simulink model "rov_property"  (Simulink 6.0)
settings: Solver=ode45  StartTime=0.0  StopTime=20  RelTol=1e-5
undefined symbols (not defined in the file): B, DQ, DQL, I, m, M, Ma, MaU, rg, T, uc1, uc2, uc3, uc4, W, xb, xg, Xudot, yb, yg, Yvdot, zb, zg, Zwdot
libraries: simulink x18, rov_design_analysis x5
(part 1 of 2)
settings Model: LastModifiedBy=c chin

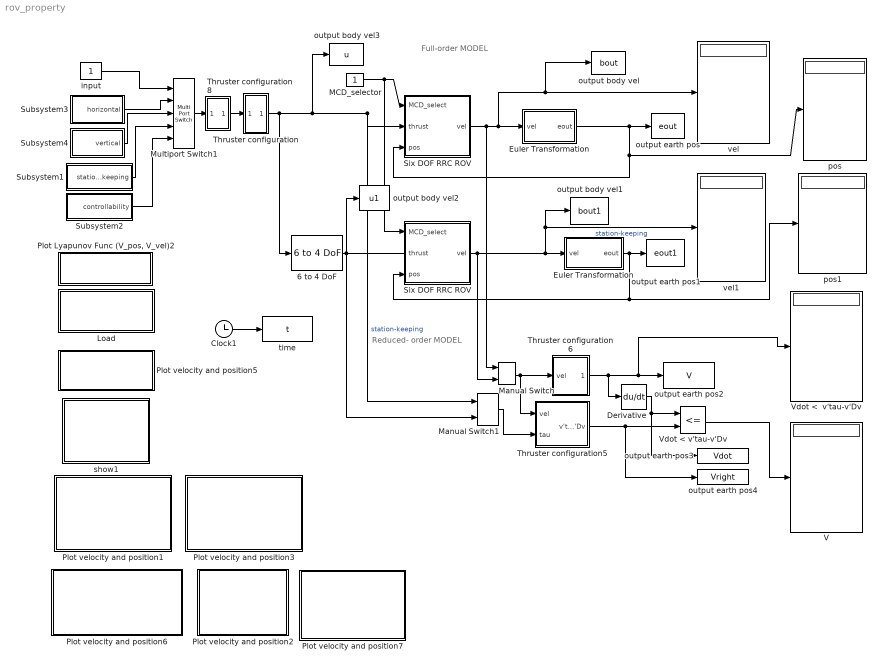
== system rov_property ==
  note: Full-order MODEL
  note: Reduced- order
      | MODEL
  " Load  " : Subsystem  AncestorBlock=|
      | rov_design_analysis/ROV Controller
      | Design
      | Applications/ Load RRCROV2 parameters
      settings: OpenFcn=|
      | clear
      | clc
      | cd c:\Matlab7\toolbox\rov_design_analysis\\mat_file ;
      | load rrcrovf;
      | cd c:\Matlab7\toolbox\rov_design_analysis\hybrid ;
      | uc1=70;uc2=70;uc3=70;uc4=70;
      mask Display: disp('Load the\n RRCROV2\n parameters')
  " Six DOF RRC ROV  " : Subsystem
      mask Display:
      | disp('ROV')
      | image(imread('/rov_design_analysis/fig/ROVRRC2.jpg'));
      | color('white');port_label('input',2,'thrust')
      | color('white');port_label('input',1,'MCD_select')
      | color('white');port_label('input',3,'pos')
      | color('white');port_label('output',1,'vel')
      | color('white');port_label('output',2,'Inv_MC')
  " Six DOF RRC ROV   " : Subsystem
      mask Display:
      | disp('ROV')
      | image(imread('/rov_design_analysis/fig/ROVRRC2.jpg'));
      | color('white');port_label('input',2,'thrust')
      | color('white');port_label('input',1,'MCD_select')
      | color('white');port_label('input',3,'pos')
      | color('white');port_label('output',1,'vel')
      | color('white');port_label('output',2,'Inv_MC')
  6 to 4 DoF : rov_design_analysis/Utilities/6 to 4 DoF
  Clock1 : Clock
      settings: Decimation=10
  Derivative : Derivative
  Euler Transformation : Subsystem  AncestorBlock=rov_design_analysis/Scope Utilities/Euler Transformation
  "Euler Transformation  " : Subsystem  AncestorBlock=rov_design_analysis/Scope Utilities/Euler Transformation
  MCD_selector : Constant
  Manual Switch : simulink/Signal Routing/Manual Switch  sw=0  action=0
  Manual Switch1 : simulink/Signal Routing/Manual Switch  sw=0  action=0
  Multiport Switch1 : MultiPortSwitch
  "Plot Lyapunov Func (V_pos, V_vel)2" : Subsystem  AncestorBlock=|
      | rov_design_analysis/ROV Controller
      | Design
      | Applications/Plot velocity and position
      settings: OpenFcn=|
      | clc
      | close all
      mask Display: disp('Close All Figure')
  Plot velocity and position1 : Subsystem  AncestorBlock=|
      | rov_design_analysis/ROV Controller
      | Design
      | Applications/Plot velocity and position
      settings: OpenFcn=|
      | clc
      | cd c:\Matlab7\toolbox\rov_design_analysis\hybrid
      | run nonlin_unique
      mask Display: disp('2a) Double-click \n to \n check \n Uniqueness/Existence \n & Continuous \n (Station)')
  Plot velocity and position2 : Subsystem  AncestorBlock=|
      | rov_design_analysis/ROV Controller
      | Design
      | Applications/Plot velocity and position
      settings: OpenFcn=|
      | clc
      | cd C:\Matlab7\toolbox\rov_design_analysis\nonlin_analysis
      | run control_analy
      mask Display: disp('3b) Double-click \n to \n check \n controllability ')
  Plot velocity and position3 : Subsystem  AncestorBlock=|
      | rov_design_analysis/ROV Controller
      | Design
      | Applications/Plot velocity and position
      settings: OpenFcn=|
      | clc
      | cd c:\Matlab7\toolbox\rov_design_analysis\hybrid
      | run nonlin_unique_plane
      mask Display: disp('2b) Double-click \n to \n check \n Uniqueness/Existence \n & Continuous \n (Vert/Hort)')
  Plot velocity and position5 : Subsystem  AncestorBlock=|
      | rov_design_analysis/ROV Controller
      | Design
      | Applications/Plot velocity and position
      settings: OpenFcn=|
      | clc
      | cd c:\Matlab7\toolbox\rov_design_analysis\hybrid
      | sim('rov_property')
      mask Display: disp('Run  SIMULINK')
  Plot velocity and position6 : Subsystem  AncestorBlock=|
      | rov_design_analysis/ROV Controller
      | Design
      | Applications/Plot velocity and position
      settings: OpenFcn=|
      | clc
      | cd C:\Matlab7\toolbox\rov_design_analysis\hybrid
      | run controllable_property
      mask Display: disp('3a) Double-click \n to \n check \n unactuated/actuated mode')
  Plot velocity and position7 : Subsystem  AncestorBlock=|
      | rov_design_analysis/ROV Controller
      | Design
      | Applications/Plot velocity and position
      settings: OpenFcn=|
      | clc
      | cd C:\Matlab7\toolbox\rov_design_analysis\hybrid
      | open controllable_property
      mask Display: disp('3c) Open \n controllability mdl')
  Subsystem1 : Subsystem
  Subsystem2 : Subsystem
  Subsystem3 : Subsystem
  Subsystem4 : Subsystem
  Thruster configuration : Subsystem
      mask Display: disp('T')
  Thruster configuration5 : Subsystem
  Thruster configuration6 : Subsystem
      mask Display:
      | disp('')
      | color('black');port_label('input',1,'vel')
      | color('black');port_label('output',1,'V')
  Thruster configuration8 : Subsystem  AncestorBlock=|
      | rov_design_analysis/ROV Controller
      | Design
      | Applications/1. Heading autopilot/Thruster
      | configuration
      mask Display: disp('F_T')
  "V " : Display
  "Vdot <  v'tau-v'Dv " : Display
  Vdot < v'tau-v'Dv : RelationalOperator  Operator=<=  LogicOutDataTypeMode=Boolean
  "input " : Constant
  output body vel : ToWorkspace  VariableName=bout  SampleTime=1  SaveFormat=Array
  output body vel1 : ToWorkspace  VariableName=bout1  SampleTime=1  SaveFormat=Array
  output body vel2 : ToWorkspace  VariableName=u1  SampleTime=1  SaveFormat=Array
  output body vel3 : ToWorkspace  VariableName=u  SampleTime=1  SaveFormat=Array
  output earth pos : ToWorkspace  VariableName=eout  SampleTime=1  SaveFormat=Array
  output earth pos1 : ToWorkspace  VariableName=eout1  SampleTime=1  SaveFormat=Array
  output earth pos2 : ToWorkspace  VariableName=V  SampleTime=1  SaveFormat=Array
  output earth pos3 : ToWorkspace  VariableName=Vdot  SampleTime=1  SaveFormat=Array
  output earth pos4 : ToWorkspace  VariableName=Vright  SampleTime=1  SaveFormat=Array
  pos : Display
  pos1 : Display
  show1 : Subsystem  AncestorBlock=|
      | rov_design_analysis/ROV Controller
      | Design
      | Applications/ Load RRCROV2 parameters
      settings: OpenFcn=|
      | clc
      | cd  c:\Matlab7\toolbox\rov_design_analysis\m_file
      | run state_coupling
      mask Display: disp('1) Open \n state-coupling \n analysis')
  time : ToWorkspace  VariableName=t  SampleTime=1  SaveFormat=Array
  vel : Display
  vel1 : Display
  wires:
  Thruster configuration/1(output force) -> output body vel3/1, Manual Switch1/1, " Six DOF RRC ROV   "/2("thrust "), 6 to 4 DoF/1  "station-keeping"
  Clock1/1 -> time/1
  Subsystem4/1(vertical) -> Multiport Switch1/3
  Subsystem3/1(horizontal) -> Multiport Switch1/2
  "input "/1 -> Multiport Switch1/1
  Subsystem1/1(station-keeping) -> Multiport Switch1/4
  Multiport Switch1/1 -> Thruster configuration8/1(input velocity)
  Thruster configuration8/1(output force) -> Thruster configuration/1(input velocity)
  Euler Transformation/1(eout) -> output earth pos/1, pos/1, " Six DOF RRC ROV   "/3("pos ")
  " Six DOF RRC ROV   "/1(vel) -> Euler Transformation/1(vel), output body vel/1, vel/1, Manual Switch/1
  Thruster configuration6/1(energy) -> Derivative/1, output earth pos2/1, "Vdot <  v'tau-v'Dv "/1
  Derivative/1 -> Vdot < v'tau-v'Dv/1, output earth pos3/1
  Thruster configuration5/1(v'tau-v'Dv) -> Vdot < v'tau-v'Dv/2, output earth pos4/1
  Manual Switch/1 -> Thruster configuration6/1(vel), Thruster configuration5/1(vel)
  Manual Switch1/1 -> Thruster configuration5/2(tau)
  Vdot < v'tau-v'Dv/1 -> "V "/1
  " Six DOF RRC ROV  "/1(vel) -> Manual Switch/2, "Euler Transformation  "/1(vel), output body vel1/1, vel1/1  "station-keeping"
  "Euler Transformation  "/1(eout) -> output earth pos1/1, pos1/1, " Six DOF RRC ROV  "/3("pos ")
  6 to 4 DoF/1 -> Manual Switch1/2, " Six DOF RRC ROV  "/2("thrust "), output body vel2/1
  MCD_selector/1 -> " Six DOF RRC ROV   "/1(MCD_select), " Six DOF RRC ROV  "/1(MCD_select)
  Subsystem2/1(controllability) -> Multiport Switch1/5

== system rov_property/ Load   ==

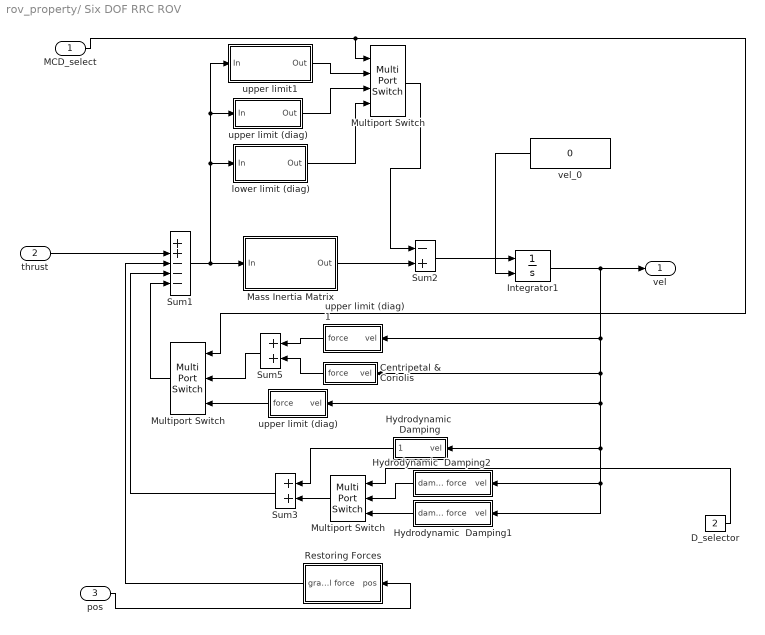
== system rov_property/ Six DOF RRC ROV   ==
  MCD_select : Inport  Port=1  LatchInput=off
  "thrust " : Inport  Port=2  LatchInput=off
  "pos " : Inport  Port=3  LatchInput=off
  Centripetal & Coriolis : Subsystem  Orientation=left  AncestorBlock=rov_design_analysis/ROV Models/1. Six DOF RRC ROV II/Centripetal & Coriolis
      mask Display: disp('C')
  D_selector : Constant  Value=2
  Hydrodynamic  Damping : Subsystem  Orientation=left
      mask Display: disp('D')
  Hydrodynamic  Damping1 : Subsystem  Orientation=left
      mask Display: disp('perturb \nDamping')
  Hydrodynamic  Damping2 : Subsystem  Orientation=left
      mask Display: disp('Zero Perturb')
  Integrator1 : Integrator  InitialConditionSource=external
  Mass Inertia Matrix : Subsystem
      mask Display: disp('inv(MRB+MA)')
  Multiport Switch : MultiPortSwitch  Inputs=3
  "Multiport Switch  " : MultiPortSwitch  Orientation=left  Inputs=2
  "Multiport Switch    " : MultiPortSwitch  Orientation=left  Inputs=2
  Restoring Forces : Subsystem  Orientation=left
      mask Display: disp('Restoring\nForce')
  Sum1 : Sum  Inputs=++---  SaturateOnIntegerOverflow=on  InputSameDT=on
  Sum2 : Sum  Inputs=-+  SaturateOnIntegerOverflow=on  InputSameDT=on
  Sum3 : Sum  Orientation=left  SaturateOnIntegerOverflow=on  InputSameDT=on
  Sum5 : Sum  Orientation=left  SaturateOnIntegerOverflow=on  InputSameDT=on
  lower limit (diag) : Subsystem
      mask Display: disp('Perturb MA')
  upper limit (diag) : Subsystem
      mask Display: disp('Perturb MA')
  "upper limit (diag)   " : Subsystem  Orientation=left
      mask Display: disp('Perturb CA')
  upper limit (diag)   1 : Subsystem  Orientation=left
      mask Display: disp('CA')
  upper limit1 : Subsystem
      mask Display: disp('Zero Perturb')
  vel_0 : Constant  Orientation=left  Value=0  OutDataTypeMode=double
  vel : Outport
  wires:
  Restoring Forces/1(gravitational force) -> Sum1/3
  "thrust "/1 -> Sum1/2
  Sum1/1 -> Mass Inertia Matrix/1(In), upper limit1/1(In), upper limit (diag)/1(In), lower limit (diag)/1(In)
  "Multiport Switch  "/1 -> Sum1/5
  "pos "/1 -> Restoring Forces/1(pos)
  Mass Inertia Matrix/1(Out) -> Sum2/2
  upper limit1/1(Out) -> Multiport Switch/2
  upper limit (diag)/1(Out) -> Multiport Switch/3
  lower limit (diag)/1(Out) -> Multiport Switch/4
  Multiport Switch/1 -> Sum2/1
  "upper limit (diag)   "/1(force) -> "Multiport Switch  "/3
  Sum5/1 -> "Multiport Switch  "/2
  Hydrodynamic  Damping1/1(damping force) -> "Multiport Switch    "/3
  Hydrodynamic  Damping2/1(damping force) -> "Multiport Switch    "/2
  Sum3/1 -> Sum1/4
  "Multiport Switch    "/1 -> Sum3/2
  Hydrodynamic  Damping/1(damping force) -> Sum3/1
  MCD_select/1 -> Multiport Switch/1, "Multiport Switch  "/1
  upper limit (diag)   1/1(force) -> Sum5/1
  Centripetal & Coriolis/1(force) -> Sum5/2
  Sum2/1 -> Integrator1/1
  Integrator1/1 -> vel/1, upper limit (diag)   1/1(vel), Centripetal & Coriolis/1(vel), Hydrodynamic  Damping/1(vel), Hydrodynamic  Damping1/1(vel), Hydrodynamic  Damping2/1(vel), "upper limit (diag)   "/1(vel)
  vel_0/1 -> Integrator1/2
  D_selector/1 -> "Multiport Switch    "/1

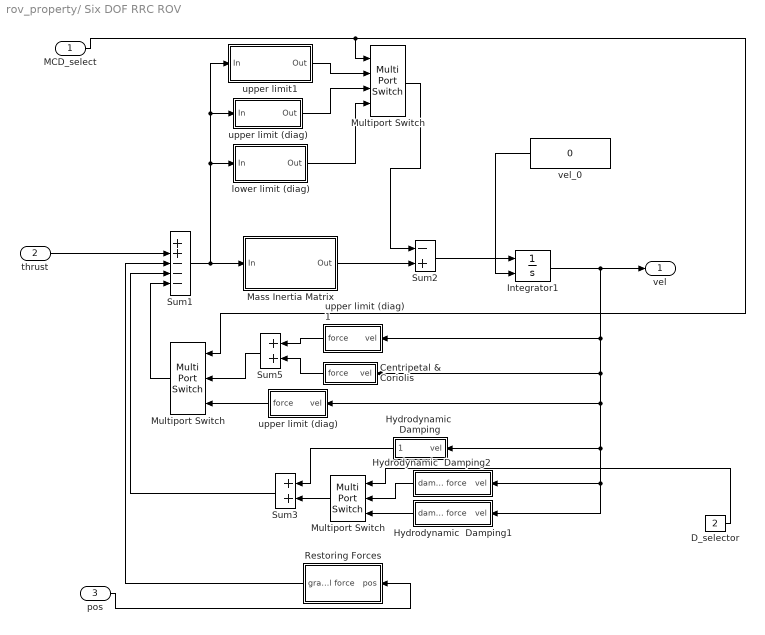
== system rov_property/ Six DOF RRC ROV    ==
  MCD_select : Inport  Port=1  LatchInput=off
  "thrust " : Inport  Port=2  LatchInput=off
  "pos " : Inport  Port=3  LatchInput=off
  Centripetal & Coriolis : Subsystem  Orientation=left  AncestorBlock=rov_design_analysis/ROV Models/1. Six DOF RRC ROV II/Centripetal & Coriolis
      mask Display: disp('C')
  D_selector : Constant  Value=2
  Hydrodynamic  Damping : Subsystem  Orientation=left
      mask Display: disp('D')
  Hydrodynamic  Damping1 : Subsystem  Orientation=left
      mask Display: disp('perturb \nDamping')
  Hydrodynamic  Damping2 : Subsystem  Orientation=left
      mask Display: disp('Zero Perturb')
  Integrator1 : Integrator  InitialConditionSource=external
  Mass Inertia Matrix : Subsystem
      mask Display: disp('inv(MRB+MA)')
  Multiport Switch : MultiPortSwitch  Inputs=3
  "Multiport Switch  " : MultiPortSwitch  Orientation=left  Inputs=2
  "Multiport Switch    " : MultiPortSwitch  Orientation=left  Inputs=2
  Restoring Forces : Subsystem  Orientation=left
      mask Display: disp('Restoring\nForce')
  Sum1 : Sum  Inputs=++---  SaturateOnIntegerOverflow=on  InputSameDT=on
  Sum2 : Sum  Inputs=-+  SaturateOnIntegerOverflow=on  InputSameDT=on
  Sum3 : Sum  Orientation=left  SaturateOnIntegerOverflow=on  InputSameDT=on
  Sum5 : Sum  Orientation=left  SaturateOnIntegerOverflow=on  InputSameDT=on
  lower limit (diag) : Subsystem
      mask Display: disp('Perturb MA')
  upper limit (diag) : Subsystem
      mask Display: disp('Perturb MA')
  "upper limit (diag)   " : Subsystem  Orientation=left
      mask Display: disp('Perturb CA')
  upper limit (diag)   1 : Subsystem  Orientation=left
      mask Display: disp('CA')
  upper limit1 : Subsystem
      mask Display: disp('Zero Perturb')
  vel_0 : Constant  Orientation=left  Value=0  OutDataTypeMode=double
  vel : Outport
  wires:
  Restoring Forces/1(gravitational force) -> Sum1/3
  "thrust "/1 -> Sum1/2
  Sum1/1 -> Mass Inertia Matrix/1(In), upper limit1/1(In), upper limit (diag)/1(In), lower limit (diag)/1(In)
  "Multiport Switch  "/1 -> Sum1/5
  "pos "/1 -> Restoring Forces/1(pos)
  Mass Inertia Matrix/1(Out) -> Sum2/2
  upper limit1/1(Out) -> Multiport Switch/2
  upper limit (diag)/1(Out) -> Multiport Switch/3
  lower limit (diag)/1(Out) -> Multiport Switch/4
  Multiport Switch/1 -> Sum2/1
  "upper limit (diag)   "/1(force) -> "Multiport Switch  "/3
  Sum5/1 -> "Multiport Switch  "/2
  Hydrodynamic  Damping1/1(damping force) -> "Multiport Switch    "/3
  Hydrodynamic  Damping2/1(damping force) -> "Multiport Switch    "/2
  Sum3/1 -> Sum1/4
  "Multiport Switch    "/1 -> Sum3/2
  Hydrodynamic  Damping/1(damping force) -> Sum3/1
  MCD_select/1 -> Multiport Switch/1, "Multiport Switch  "/1
  upper limit (diag)   1/1(force) -> Sum5/1
  Centripetal & Coriolis/1(force) -> Sum5/2
  Sum2/1 -> Integrator1/1
  Integrator1/1 -> vel/1, upper limit (diag)   1/1(vel), Centripetal & Coriolis/1(vel), Hydrodynamic  Damping/1(vel), Hydrodynamic  Damping1/1(vel), Hydrodynamic  Damping2/1(vel), "upper limit (diag)   "/1(vel)
  vel_0/1 -> Integrator1/2
  D_selector/1 -> "Multiport Switch    "/1

== system rov_property/Euler Transformation ==
  vel : Inport  Port=1  LatchInput=off
  1/s : Subsystem
  Demux : Demux  Outputs=2
  Demux1 : Demux  Outputs=2
  Mux1 : Mux  Inputs=2
  Terminator : Terminator
  Transformation matrix R : Subsystem
      mask Display: disp('Transformation R')
  Transformation matrix T : Subsystem
      mask Display: disp('Transformation T')
  eout : Outport  InitialOutput=0
  wires:
  Mux1/1 -> 1/s/1(In1)
  1/s/1(Out1) -> Demux1/1, eout/1
  Demux/2 -> Transformation matrix R/1(angular body  velocity)
  Demux/1 -> Transformation matrix T/1(translational body velocity)
  vel/1 -> Demux/1
  Demux1/2 -> Transformation matrix T/2(angular position), Transformation matrix R/2(angular position)
  Transformation matrix R/1(angular earth velocity) -> Mux1/2
  Transformation matrix T/1(translational earth velocity) -> Mux1/1
  Demux1/1 -> Terminator/1

== system rov_property/Euler Transformation   ==
  vel : Inport  Port=1  LatchInput=off
  1/s : Subsystem
  Demux : Demux  Outputs=2
  Demux1 : Demux  Outputs=2
  Mux1 : Mux  Inputs=2
  Terminator : Terminator
  Transformation matrix R : Subsystem
      mask Display: disp('Transformation R')
  Transformation matrix T : Subsystem
      mask Display: disp('Transformation T')
  eout : Outport  InitialOutput=0
  wires:
  Mux1/1 -> 1/s/1(In1)
  1/s/1(Out1) -> Demux1/1, eout/1
  Demux/2 -> Transformation matrix R/1(angular body  velocity)
  Demux/1 -> Transformation matrix T/1(translational body velocity)
  vel/1 -> Demux/1
  Demux1/2 -> Transformation matrix T/2(angular position), Transformation matrix R/2(angular position)
  Transformation matrix R/1(angular earth velocity) -> Mux1/2
  Transformation matrix T/1(translational earth velocity) -> Mux1/1
  Demux1/1 -> Terminator/1

== system rov_property/Plot Lyapunov Func (V_pos, V_vel)2 ==

== system rov_property/Plot velocity and position1 ==

== system rov_property/Plot velocity and position2 ==

== system rov_property/Plot velocity and position3 ==

== system rov_property/Plot velocity and position5 ==

== system rov_property/Plot velocity and position6 ==

== system rov_property/Plot velocity and position7 ==

== system rov_property/Subsystem1 ==
  Mux1 : Mux
  uc{1..4} (4 alike) : Step  Time=0  After=70  SampleTime=0
  station-keeping : Outport
  wires:
  uc2/1 -> Mux1/2
  uc1/1 -> Mux1/1
  uc3/1 -> Mux1/3
  uc4/1 -> Mux1/4
  Mux1/1 -> station-keeping/1

== system rov_property/Subsystem2 ==
  Constant1 : Constant  Value=uc1
  Constant2 : Constant  Value=uc2
  Constant3 : Constant  Value=uc3
  Constant4 : Constant  Value=uc4
  Mux1 : Mux
  controllability : Outport
  wires:
  Mux1/1 -> controllability/1
  Constant1/1 -> Mux1/1
  Constant2/1 -> Mux1/2
  Constant3/1 -> Mux1/3
  Constant4/1 -> Mux1/4

== system rov_property/Subsystem3 ==
  Mux1 : Mux
  u1 : Step  Time=0  After=70  SampleTime=0
  u2 : Step  Time=0  After=70  SampleTime=0
  u3 : Step  Time=0  After=0  SampleTime=0
  u4 : Step  Time=0  After=0  SampleTime=0
  horizontal : Outport
  wires:
  u2/1 -> Mux1/2
  u1/1 -> Mux1/1
  u3/1 -> Mux1/3
  Mux1/1 -> horizontal/1
  u4/1 -> Mux1/4

== system rov_property/Subsystem4 ==
  Mux1 : Mux
  u1 : Step  Time=0  After=0  SampleTime=0
  u2 : Step  Time=0  After=0  SampleTime=0
  u3 : Step  Time=0  After=70  SampleTime=0
  u4 : Step  Time=0  After=70  SampleTime=0
  vertical : Outport
  wires:
  u2/1 -> Mux1/2
  u1/1 -> Mux1/1
  u3/1 -> Mux1/3
  u4/1 -> Mux1/4
  Mux1/1 -> vertical/1

== system rov_property/Thruster configuration ==
  input velocity : Inport  Orientation=up  Port=1  LatchInput=off
  Thruster Matrix : Gain  Gain=T  Multiplication=Matrix(K*u)  SaturateOnIntegerOverflow=on
  output force : Outport  InitialOutput=0
  wires:
  input velocity/1 -> Thruster Matrix/1
  Thruster Matrix/1 -> output force/1

== system rov_property/Thruster configuration5 ==
  vel : Inport  Port=1  LatchInput=off
  tau : Inport  Port=2  LatchInput=off
  D : Gain  Gain=DQL  Multiplication=Matrix(K*u)  SaturateOnIntegerOverflow=on
  Math Function : Math  Operator=square  SaturateOnIntegerOverflow=on
  Subtract : Sum  Inputs=-+  OutScaling=2^-10
  "v'tau " : Product  RndMeth=Zero
  v'tau-v'Dv : Outport  InitialOutput=0
  wires:
  vel/1 -> "v'tau "/1, Math Function/1
  "v'tau "/1 -> Subtract/2
  tau/1 -> "v'tau "/2
  Math Function/1 -> D/1
  D/1 -> Subtract/1
  Subtract/1 -> v'tau-v'Dv/1

== system rov_property/Thruster configuration6 ==
  vel : Inport  Port=1  LatchInput=off
  Math Function : Math  Operator=square  SaturateOnIntegerOverflow=on
  Thruster Matrix : Gain  Gain=1/2*M  Multiplication=Matrix(K*u)  SaturateOnIntegerOverflow=on
  energy : Outport  InitialOutput=0
  wires:
  vel/1 -> Math Function/1
  Math Function/1 -> Thruster Matrix/1
  Thruster Matrix/1 -> energy/1

== system rov_property/Thruster configuration8 ==
  input velocity : Inport  Orientation=up  Port=1  LatchInput=off
  3. propeller with motor characteristics - 1DoF (no account for ua,up){,1..3} (4 alike) : rov_design_analysis/Propeller Models/3. propeller with motor characteristics - 1DoF (no account for ua,up)
  Demux : Demux
  Mux1 : Mux
  output force : Outport  InitialOutput=0
  wires:
  3. propeller with motor characteristics - 1DoF (no account for ua,up)/1 -> Mux1/1
  3. propeller with motor characteristics - 1DoF (no account for ua,up)1/1 -> Mux1/2
  3. propeller with motor characteristics - 1DoF (no account for ua,up)2/1 -> Mux1/3
  3. propeller with motor characteristics - 1DoF (no account for ua,up)3/1 -> Mux1/4
  Mux1/1 -> output force/1
  input velocity/1 -> Demux/1
  Demux/1 -> 3. propeller with motor characteristics - 1DoF (no account for ua,up)/1
  Demux/2 -> 3. propeller with motor characteristics - 1DoF (no account for ua,up)1/1
  Demux/3 -> 3. propeller with motor characteristics - 1DoF (no account for ua,up)2/1
  Demux/4 -> 3. propeller with motor characteristics - 1DoF (no account for ua,up)3/1

== system rov_property/show1 ==

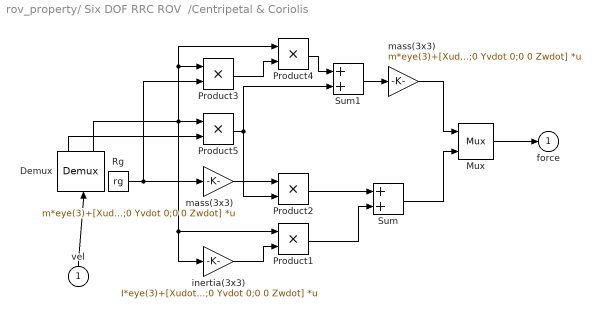
== system rov_property/ Six DOF RRC ROV  /Centripetal & Coriolis ==
  vel : Inport  Orientation=up  Port=1  LatchInput=off
  Demux : Demux  Orientation=up  Outputs=2
  Mux : Mux  Inputs=2
  Product{1..5} (5 alike) : Product  SaturateOnIntegerOverflow=on  RndMeth=Zero  InputSameDT=on
  Rg : Constant  Value=rg
  Sum : Sum  SaturateOnIntegerOverflow=on  InputSameDT=on
  Sum1 : Sum  SaturateOnIntegerOverflow=on  InputSameDT=on
  inertia(3x3) : Gain  Gain=I*eye(3)+[Xudot 0 0;0 Yvdot 0;0 0 Zwdot]  Multiplication=Matrix(K*u)  SaturateOnIntegerOverflow=on
  "mass(3x3) " : Gain  Gain=m*eye(3)+[Xudot 0 0;0 Yvdot 0;0 0 Zwdot]  Multiplication=Matrix(K*u)  SaturateOnIntegerOverflow=on
  "mass(3x3)   " : Gain  Gain=m*eye(3)+[Xudot 0 0;0 Yvdot 0;0 0 Zwdot]  Multiplication=Matrix(K*u)  SaturateOnIntegerOverflow=on
  force : Outport  InitialOutput=0
  wires:
  Product1/1 -> Sum/2
  "mass(3x3)   "/1 -> Product2/1
  Product2/1 -> Sum/1
  Rg/1 -> Product3/2, "mass(3x3)   "/1
  Product3/1 -> Product4/2
  Product4/1 -> Sum1/1
  Product5/1 -> Product2/2, Sum1/2
  Sum1/1 -> "mass(3x3) "/1
  Demux/2 -> Product5/1, Product3/1, Product4/1, Product1/1, inertia(3x3)/1
  Demux/1 -> Product5/2
  vel/1 -> Demux/1
  inertia(3x3)/1 -> Product1/2
  "mass(3x3) "/1 -> Mux/1
  Sum/1 -> Mux/2
  Mux/1 -> force/1

== system rov_property/ Six DOF RRC ROV  /Hydrodynamic  Damping ==
  vel : Inport  Port=1  LatchInput=off
  D linear : Gain  Gain=-diag(DQL)  SaturateOnIntegerOverflow=on
  damping force : Outport  InitialOutput=0
  wires:
  vel/1 -> D linear/1
  D linear/1 -> damping force/1

== system rov_property/ Six DOF RRC ROV  /Hydrodynamic  Damping1 ==
  vel : Inport  Port=1  LatchInput=off
  D quadratic : Gain  Gain=-diag(DQ)  SaturateOnIntegerOverflow=on
  Product : Product  SaturateOnIntegerOverflow=on  RndMeth=Zero  InputSameDT=on
  |u| : Abs  SaturateOnIntegerOverflow=on
  damping force : Outport  InitialOutput=0
  wires:
  Product/1 -> D quadratic/1
  vel/1 -> Product/1, |u|/1
  |u|/1 -> Product/2
  D quadratic/1 -> damping force/1

== system rov_property/ Six DOF RRC ROV  /Hydrodynamic  Damping2 ==
  vel : Inport  Port=1  LatchInput=off
  D quadratic : Gain  Gain=0  SaturateOnIntegerOverflow=on
  damping force : Outport  InitialOutput=0
  wires:
  D quadratic/1 -> damping force/1
  vel/1 -> D quadratic/1

== system rov_property/ Six DOF RRC ROV  /Mass Inertia Matrix ==
  In : Inport  Port=1  LatchInput=off
  inverse M : Gain  Gain=inv(M-Ma)  Multiplication=Matrix(K*u)  SaturateOnIntegerOverflow=on
  Out : Outport
  wires:
  inverse M/1 -> Out/1
  In/1 -> inverse M/1

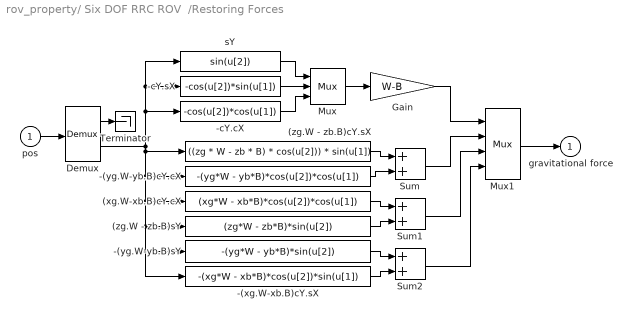
== system rov_property/ Six DOF RRC ROV  /Restoring Forces ==
  pos : Inport  Port=1  LatchInput=off
  (xg.W-xb.B)cY.cX : Fcn  Expr=(xg*W - xb*B)*cos(u[2])*cos(u[1])
  (zg.W - zb.B)cY.sX : Fcn  Expr=((zg * W - zb * B) * cos(u[2])) * sin(u[1])
  (zg.W - zb.B)sY : Fcn  Expr=(zg*W - zb*B)*sin(u[2])
  -(xg.W-xb.B)cY.sX : Fcn  Expr=-(xg*W - xb*B)*cos(u[2])*sin(u[1])
  -(yg.W-yb.B)cY.cX : Fcn  Expr=-(yg*W - yb*B)*cos(u[2])*cos(u[1])
  -(yg.W-yb.B)sY : Fcn  Expr=-(yg*W - yb*B)*sin(u[2])
  -cY.cX : Fcn  Expr=-cos(u[2])*cos(u[1])
  -cY.sX : Fcn  Expr=-cos(u[2])*sin(u[1])
  Demux : Demux  Outputs=2
  Gain : Gain  Gain=W-B  SaturateOnIntegerOverflow=on
  Mux : Mux  Inputs=3
  Mux1 : Mux
  Sum : Sum  SaturateOnIntegerOverflow=on  InputSameDT=on
  Sum1 : Sum  SaturateOnIntegerOverflow=on  InputSameDT=on
  Sum2 : Sum  SaturateOnIntegerOverflow=on  InputSameDT=on
  Terminator : Terminator
  sY : Fcn  Expr=sin(u[2])
  gravitational force : Outport  InitialOutput=0
  wires:
  Sum2/1 -> Mux1/4
  -(yg.W-yb.B)sY/1 -> Sum2/1
  -(xg.W-xb.B)cY.sX/1 -> Sum2/2
  Sum1/1 -> Mux1/3
  (xg.W-xb.B)cY.cX/1 -> Sum1/1
  (zg.W - zb.B)sY/1 -> Sum1/2
  Sum/1 -> Mux1/2
  (zg.W - zb.B)cY.sX/1 -> Sum/1
  -(yg.W-yb.B)cY.cX/1 -> Sum/2
  Gain/1 -> Mux1/1
  Mux/1 -> Gain/1
  -cY.cX/1 -> Mux/3
  -cY.sX/1 -> Mux/2
  sY/1 -> Mux/1
  Mux1/1 -> gravitational force/1
  Demux/2 -> -(xg.W-xb.B)cY.sX/1, -(yg.W-yb.B)sY/1, (zg.W - zb.B)sY/1, (xg.W-xb.B)cY.cX/1, -(yg.W-yb.B)cY.cX/1, (zg.W - zb.B)cY.sX/1, sY/1, -cY.sX/1, -cY.cX/1
  Demux/1 -> Terminator/1
  pos/1 -> Demux/1

== system rov_property/ Six DOF RRC ROV  /lower limit (diag) ==
  In : Inport  Port=1  LatchInput=off
  inverse M : Gain  Gain=-diag([21.1403-21.0981 51.7012-51.0026 92.451-91.837 3.6191-3.576 2.6427-2.7687 2.3033-2.3493])  Multiplication=Matrix(K*u)  SaturateOnIntegerOverflow=on
  Out : Outport
  wires:
  inverse M/1 -> Out/1
  In/1 -> inverse M/1

== system rov_property/ Six DOF RRC ROV  /upper limit (diag) ==
  In : Inport  Port=1  LatchInput=off
  inverse M : Gain  Gain=-diag([21.724-21.1403 51.7013-51.7012 94.3-92.451 4.2176-3.6191 7.1148-2.6427 4.7673-2.3033])  Multiplication=Matrix(K*u)  SaturateOnIntegerOverflow=on
  Out : Outport
  wires:
  inverse M/1 -> Out/1
  In/1 -> inverse M/1

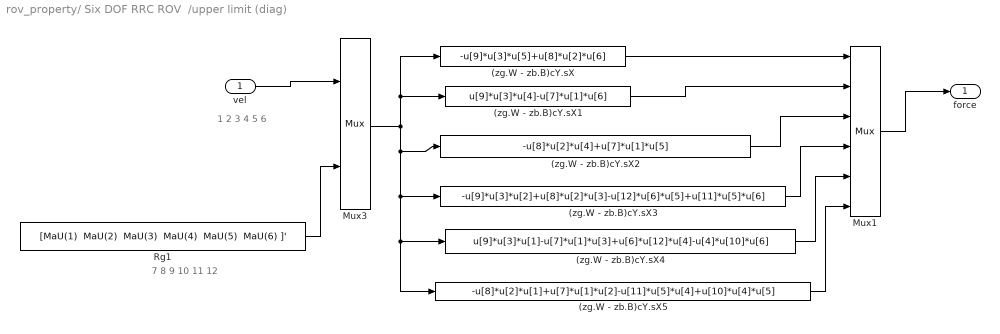
== system rov_property/ Six DOF RRC ROV  /upper limit (diag)    ==
  note: 7 8 9 10 11 12
  note: 1 2 3 4 5 6
  vel : Inport  Port=1  LatchInput=off
  (zg.W - zb.B)cY.sX : Fcn  Expr=-u[9]*u[3]*u[5]+u[8]*u[2]*u[6]
  (zg.W - zb.B)cY.sX1 : Fcn  Expr=u[9]*u[3]*u[4]-u[7]*u[1]*u[6]
  (zg.W - zb.B)cY.sX2 : Fcn  Expr=-u[8]*u[2]*u[4]+u[7]*u[1]*u[5]
  (zg.W - zb.B)cY.sX3 : Fcn  Expr=-u[9]*u[3]*u[2]+u[8]*u[2]*u[3]-u[12]*u[6]*u[5]+u[11]*u[5]*u[6]
  (zg.W - zb.B)cY.sX4 : Fcn  Expr=u[9]*u[3]*u[1]-u[7]*u[1]*u[3]+u[6]*u[12]*u[4]-u[4]*u[10]*u[6]
  (zg.W - zb.B)cY.sX5 : Fcn  Expr=-u[8]*u[2]*u[1]+u[7]*u[1]*u[2]-u[11]*u[5]*u[4]+u[10]*u[4]*u[5]
  Mux1 : Mux  Inputs=6
  Mux3 : Mux  Inputs=2
  Rg1 : Constant  Value="[MaU(1)  MaU(2)  MaU(3)  MaU(4)  MaU(5)  MaU(6) ]'"
  force : Outport
  wires:
  Mux1/1 -> force/1
  (zg.W - zb.B)cY.sX/1 -> Mux1/1
  (zg.W - zb.B)cY.sX1/1 -> Mux1/2
  (zg.W - zb.B)cY.sX2/1 -> Mux1/3
  (zg.W - zb.B)cY.sX3/1 -> Mux1/4
  (zg.W - zb.B)cY.sX4/1 -> Mux1/5
  (zg.W - zb.B)cY.sX5/1 -> Mux1/6
  vel/1 -> Mux3/1
  Rg1/1 -> Mux3/2
  Mux3/1 -> (zg.W - zb.B)cY.sX/1, (zg.W - zb.B)cY.sX1/1, (zg.W - zb.B)cY.sX4/1, (zg.W - zb.B)cY.sX5/1, (zg.W - zb.B)cY.sX3/1, (zg.W - zb.B)cY.sX2/1

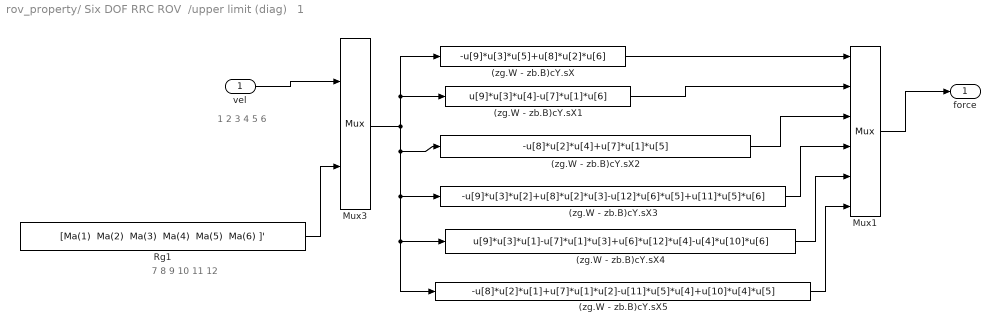
== system rov_property/ Six DOF RRC ROV  /upper limit (diag)   1 ==
  note: 7 8 9 10 11 12
  note: 1 2 3 4 5 6
  vel : Inport  Port=1  LatchInput=off
  (zg.W - zb.B)cY.sX : Fcn  Expr=-u[9]*u[3]*u[5]+u[8]*u[2]*u[6]
  (zg.W - zb.B)cY.sX1 : Fcn  Expr=u[9]*u[3]*u[4]-u[7]*u[1]*u[6]
  (zg.W - zb.B)cY.sX2 : Fcn  Expr=-u[8]*u[2]*u[4]+u[7]*u[1]*u[5]
  (zg.W - zb.B)cY.sX3 : Fcn  Expr=-u[9]*u[3]*u[2]+u[8]*u[2]*u[3]-u[12]*u[6]*u[5]+u[11]*u[5]*u[6]
  (zg.W - zb.B)cY.sX4 : Fcn  Expr=u[9]*u[3]*u[1]-u[7]*u[1]*u[3]+u[6]*u[12]*u[4]-u[4]*u[10]*u[6]
  (zg.W - zb.B)cY.sX5 : Fcn  Expr=-u[8]*u[2]*u[1]+u[7]*u[1]*u[2]-u[11]*u[5]*u[4]+u[10]*u[4]*u[5]
  Mux1 : Mux  Inputs=6
  Mux3 : Mux  Inputs=2
  Rg1 : Constant  Value="[Ma(1)  Ma(2)  Ma(3)  Ma(4)  Ma(5)  Ma(6) ]'"
  force : Outport
  wires:
  Mux1/1 -> force/1
  (zg.W - zb.B)cY.sX/1 -> Mux1/1
  (zg.W - zb.B)cY.sX1/1 -> Mux1/2
  (zg.W - zb.B)cY.sX2/1 -> Mux1/3
  (zg.W - zb.B)cY.sX3/1 -> Mux1/4
  (zg.W - zb.B)cY.sX4/1 -> Mux1/5
  (zg.W - zb.B)cY.sX5/1 -> Mux1/6
  vel/1 -> Mux3/1
  Rg1/1 -> Mux3/2
  Mux3/1 -> (zg.W - zb.B)cY.sX/1, (zg.W - zb.B)cY.sX1/1, (zg.W - zb.B)cY.sX4/1, (zg.W - zb.B)cY.sX5/1, (zg.W - zb.B)cY.sX3/1, (zg.W - zb.B)cY.sX2/1

== system rov_property/ Six DOF RRC ROV  /upper limit1 ==
  In : Inport  Port=1  LatchInput=off
  inverse M : Gain  Gain=0  Multiplication=Matrix(K*u)  SaturateOnIntegerOverflow=on
  Out : Outport
  wires:
  inverse M/1 -> Out/1
  In/1 -> inverse M/1

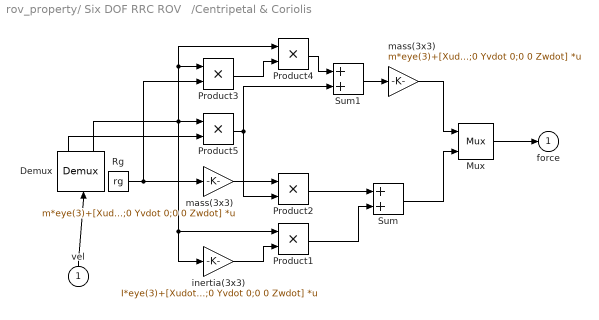
== system rov_property/ Six DOF RRC ROV   /Centripetal & Coriolis ==
  vel : Inport  Orientation=up  Port=1  LatchInput=off
  Demux : Demux  Orientation=up  Outputs=2
  Mux : Mux  Inputs=2
  Product{1..5} (5 alike) : Product  SaturateOnIntegerOverflow=on  RndMeth=Zero  InputSameDT=on
  Rg : Constant  Value=rg
  Sum : Sum  SaturateOnIntegerOverflow=on  InputSameDT=on
  Sum1 : Sum  SaturateOnIntegerOverflow=on  InputSameDT=on
  inertia(3x3) : Gain  Gain=I*eye(3)+[Xudot 0 0;0 Yvdot 0;0 0 Zwdot]  Multiplication=Matrix(K*u)  SaturateOnIntegerOverflow=on
  "mass(3x3) " : Gain  Gain=m*eye(3)+[Xudot 0 0;0 Yvdot 0;0 0 Zwdot]  Multiplication=Matrix(K*u)  SaturateOnIntegerOverflow=on
  "mass(3x3)   " : Gain  Gain=m*eye(3)+[Xudot 0 0;0 Yvdot 0;0 0 Zwdot]  Multiplication=Matrix(K*u)  SaturateOnIntegerOverflow=on
  force : Outport  InitialOutput=0
  wires:
  Product1/1 -> Sum/2
  "mass(3x3)   "/1 -> Product2/1
  Product2/1 -> Sum/1
  Rg/1 -> Product3/2, "mass(3x3)   "/1
  Product3/1 -> Product4/2
  Product4/1 -> Sum1/1
  Product5/1 -> Product2/2, Sum1/2
  Sum1/1 -> "mass(3x3) "/1
  Demux/2 -> Product5/1, Product3/1, Product4/1, Product1/1, inertia(3x3)/1
  Demux/1 -> Product5/2
  vel/1 -> Demux/1
  inertia(3x3)/1 -> Product1/2
  "mass(3x3) "/1 -> Mux/1
  Sum/1 -> Mux/2
  Mux/1 -> force/1

== system rov_property/ Six DOF RRC ROV   /Hydrodynamic  Damping ==
  vel : Inport  Port=1  LatchInput=off
  D linear : Gain  Gain=-diag(DQL)  SaturateOnIntegerOverflow=on
  damping force : Outport  InitialOutput=0
  wires:
  vel/1 -> D linear/1
  D linear/1 -> damping force/1

== system rov_property/ Six DOF RRC ROV   /Hydrodynamic  Damping1 ==
  vel : Inport  Port=1  LatchInput=off
  D quadratic : Gain  Gain=-diag(DQ)  SaturateOnIntegerOverflow=on
  Product : Product  SaturateOnIntegerOverflow=on  RndMeth=Zero  InputSameDT=on
  |u| : Abs  SaturateOnIntegerOverflow=on
  damping force : Outport  InitialOutput=0
  wires:
  Product/1 -> D quadratic/1
  vel/1 -> Product/1, |u|/1
  |u|/1 -> Product/2
  D quadratic/1 -> damping force/1

== system rov_property/ Six DOF RRC ROV   /Hydrodynamic  Damping2 ==
  vel : Inport  Port=1  LatchInput=off
  D quadratic : Gain  Gain=0  SaturateOnIntegerOverflow=on
  damping force : Outport  InitialOutput=0
  wires:
  D quadratic/1 -> damping force/1
  vel/1 -> D quadratic/1

== system rov_property/ Six DOF RRC ROV   /Mass Inertia Matrix ==
  In : Inport  Port=1  LatchInput=off
  inverse M : Gain  Gain=inv(M-Ma)  Multiplication=Matrix(K*u)  SaturateOnIntegerOverflow=on
  Out : Outport
  wires:
  inverse M/1 -> Out/1
  In/1 -> inverse M/1

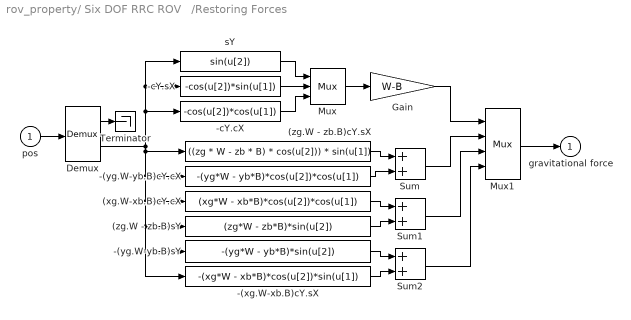
== system rov_property/ Six DOF RRC ROV   /Restoring Forces ==
  pos : Inport  Port=1  LatchInput=off
  (xg.W-xb.B)cY.cX : Fcn  Expr=(xg*W - xb*B)*cos(u[2])*cos(u[1])
  (zg.W - zb.B)cY.sX : Fcn  Expr=((zg * W - zb * B) * cos(u[2])) * sin(u[1])
  (zg.W - zb.B)sY : Fcn  Expr=(zg*W - zb*B)*sin(u[2])
  -(xg.W-xb.B)cY.sX : Fcn  Expr=-(xg*W - xb*B)*cos(u[2])*sin(u[1])
  -(yg.W-yb.B)cY.cX : Fcn  Expr=-(yg*W - yb*B)*cos(u[2])*cos(u[1])
  -(yg.W-yb.B)sY : Fcn  Expr=-(yg*W - yb*B)*sin(u[2])
  -cY.cX : Fcn  Expr=-cos(u[2])*cos(u[1])
  -cY.sX : Fcn  Expr=-cos(u[2])*sin(u[1])
  Demux : Demux  Outputs=2
  Gain : Gain  Gain=W-B  SaturateOnIntegerOverflow=on
  Mux : Mux  Inputs=3
  Mux1 : Mux
  Sum : Sum  SaturateOnIntegerOverflow=on  InputSameDT=on
  Sum1 : Sum  SaturateOnIntegerOverflow=on  InputSameDT=on
  Sum2 : Sum  SaturateOnIntegerOverflow=on  InputSameDT=on
  Terminator : Terminator
  sY : Fcn  Expr=sin(u[2])
  gravitational force : Outport  InitialOutput=0
  wires:
  Sum2/1 -> Mux1/4
  -(yg.W-yb.B)sY/1 -> Sum2/1
  -(xg.W-xb.B)cY.sX/1 -> Sum2/2
  Sum1/1 -> Mux1/3
  (xg.W-xb.B)cY.cX/1 -> Sum1/1
  (zg.W - zb.B)sY/1 -> Sum1/2
  Sum/1 -> Mux1/2
  (zg.W - zb.B)cY.sX/1 -> Sum/1
  -(yg.W-yb.B)cY.cX/1 -> Sum/2
  Gain/1 -> Mux1/1
  Mux/1 -> Gain/1
  -cY.cX/1 -> Mux/3
  -cY.sX/1 -> Mux/2
  sY/1 -> Mux/1
  Mux1/1 -> gravitational force/1
  Demux/2 -> -(xg.W-xb.B)cY.sX/1, -(yg.W-yb.B)sY/1, (zg.W - zb.B)sY/1, (xg.W-xb.B)cY.cX/1, -(yg.W-yb.B)cY.cX/1, (zg.W - zb.B)cY.sX/1, sY/1, -cY.sX/1, -cY.cX/1
  Demux/1 -> Terminator/1
  pos/1 -> Demux/1

== system rov_property/ Six DOF RRC ROV   /lower limit (diag) ==
  In : Inport  Port=1  LatchInput=off
  inverse M : Gain  Gain=-diag([21.1403-21.0981 51.7012-51.0026 92.451-91.837 3.6191-3.576 2.6427-2.7687 2.3033-2.3493])  Multiplication=Matrix(K*u)  SaturateOnIntegerOverflow=on
  Out : Outport
  wires:
  inverse M/1 -> Out/1
  In/1 -> inverse M/1

== system rov_property/ Six DOF RRC ROV   /upper limit (diag) ==
  In : Inport  Port=1  LatchInput=off
  inverse M : Gain  Gain=-diag([21.724-21.1403 51.7013-51.7012 94.3-92.451 4.2176-3.6191 7.1148-2.6427 4.7673-2.3033])  Multiplication=Matrix(K*u)  SaturateOnIntegerOverflow=on
  Out : Outport
  wires:
  inverse M/1 -> Out/1
  In/1 -> inverse M/1

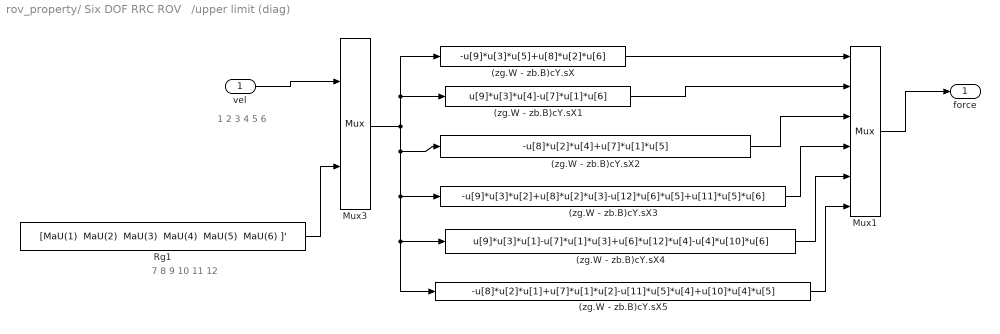
== system rov_property/ Six DOF RRC ROV   /upper limit (diag)    ==
  note: 7 8 9 10 11 12
  note: 1 2 3 4 5 6
  vel : Inport  Port=1  LatchInput=off
  (zg.W - zb.B)cY.sX : Fcn  Expr=-u[9]*u[3]*u[5]+u[8]*u[2]*u[6]
  (zg.W - zb.B)cY.sX1 : Fcn  Expr=u[9]*u[3]*u[4]-u[7]*u[1]*u[6]
  (zg.W - zb.B)cY.sX2 : Fcn  Expr=-u[8]*u[2]*u[4]+u[7]*u[1]*u[5]
  (zg.W - zb.B)cY.sX3 : Fcn  Expr=-u[9]*u[3]*u[2]+u[8]*u[2]*u[3]-u[12]*u[6]*u[5]+u[11]*u[5]*u[6]
  (zg.W - zb.B)cY.sX4 : Fcn  Expr=u[9]*u[3]*u[1]-u[7]*u[1]*u[3]+u[6]*u[12]*u[4]-u[4]*u[10]*u[6]
  (zg.W - zb.B)cY.sX5 : Fcn  Expr=-u[8]*u[2]*u[1]+u[7]*u[1]*u[2]-u[11]*u[5]*u[4]+u[10]*u[4]*u[5]
  Mux1 : Mux  Inputs=6
  Mux3 : Mux  Inputs=2
  Rg1 : Constant  Value="[MaU(1)  MaU(2)  MaU(3)  MaU(4)  MaU(5)  MaU(6) ]'"
  force : Outport
  wires:
  Mux1/1 -> force/1
  (zg.W - zb.B)cY.sX/1 -> Mux1/1
  (zg.W - zb.B)cY.sX1/1 -> Mux1/2
  (zg.W - zb.B)cY.sX2/1 -> Mux1/3
  (zg.W - zb.B)cY.sX3/1 -> Mux1/4
  (zg.W - zb.B)cY.sX4/1 -> Mux1/5
  (zg.W - zb.B)cY.sX5/1 -> Mux1/6
  vel/1 -> Mux3/1
  Rg1/1 -> Mux3/2
  Mux3/1 -> (zg.W - zb.B)cY.sX/1, (zg.W - zb.B)cY.sX1/1, (zg.W - zb.B)cY.sX4/1, (zg.W - zb.B)cY.sX5/1, (zg.W - zb.B)cY.sX3/1, (zg.W - zb.B)cY.sX2/1

== system rov_property/ Six DOF RRC ROV   /upper limit (diag)   1 ==
  note: 7 8 9 10 11 12
  note: 1 2 3 4 5 6
  vel : Inport  Port=1  LatchInput=off
  (zg.W - zb.B)cY.sX : Fcn  Expr=-u[9]*u[3]*u[5]+u[8]*u[2]*u[6]
  (zg.W - zb.B)cY.sX1 : Fcn  Expr=u[9]*u[3]*u[4]-u[7]*u[1]*u[6]
  (zg.W - zb.B)cY.sX2 : Fcn  Expr=-u[8]*u[2]*u[4]+u[7]*u[1]*u[5]
  (zg.W - zb.B)cY.sX3 : Fcn  Expr=-u[9]*u[3]*u[2]+u[8]*u[2]*u[3]-u[12]*u[6]*u[5]+u[11]*u[5]*u[6]
  (zg.W - zb.B)cY.sX4 : Fcn  Expr=u[9]*u[3]*u[1]-u[7]*u[1]*u[3]+u[6]*u[12]*u[4]-u[4]*u[10]*u[6]
  (zg.W - zb.B)cY.sX5 : Fcn  Expr=-u[8]*u[2]*u[1]+u[7]*u[1]*u[2]-u[11]*u[5]*u[4]+u[10]*u[4]*u[5]
  Mux1 : Mux  Inputs=6
  Mux3 : Mux  Inputs=2
  Rg1 : Constant  Value="[Ma(1)  Ma(2)  Ma(3)  Ma(4)  Ma(5)  Ma(6) ]'"
  force : Outport
  wires:
  Mux1/1 -> force/1
  (zg.W - zb.B)cY.sX/1 -> Mux1/1
  (zg.W - zb.B)cY.sX1/1 -> Mux1/2
  (zg.W - zb.B)cY.sX2/1 -> Mux1/3
  (zg.W - zb.B)cY.sX3/1 -> Mux1/4
  (zg.W - zb.B)cY.sX4/1 -> Mux1/5
  (zg.W - zb.B)cY.sX5/1 -> Mux1/6
  vel/1 -> Mux3/1
  Rg1/1 -> Mux3/2
  Mux3/1 -> (zg.W - zb.B)cY.sX/1, (zg.W - zb.B)cY.sX1/1, (zg.W - zb.B)cY.sX4/1, (zg.W - zb.B)cY.sX5/1, (zg.W - zb.B)cY.sX3/1, (zg.W - zb.B)cY.sX2/1

== system rov_property/ Six DOF RRC ROV   /upper limit1 ==
  In : Inport  Port=1  LatchInput=off
  inverse M : Gain  Gain=0  Multiplication=Matrix(K*u)  SaturateOnIntegerOverflow=on
  Out : Outport
  wires:
  inverse M/1 -> Out/1
  In/1 -> inverse M/1

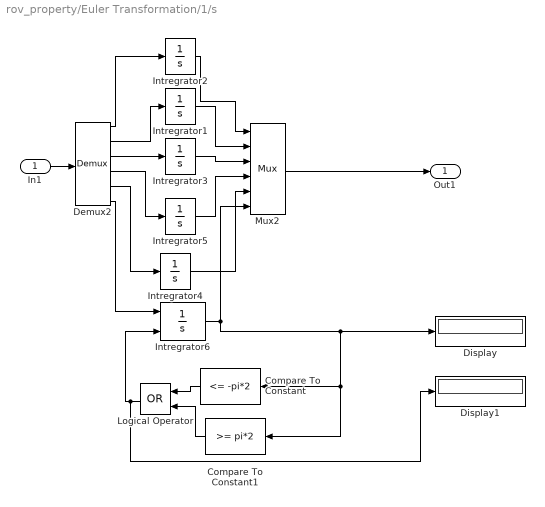
== system rov_property/Euler Transformation/1/s ==
  In1 : Inport  Port=1  LatchInput=off
  Compare To Constant : simulink/Logic and Bit Operations/Compare To Constant  Orientation=left  relop=<=  const=-pi*2  LogicOutDataTypeMode=boolean
  Compare To Constant1 : simulink/Logic and Bit Operations/Compare To Constant  Orientation=left  relop=>=  const=pi*2  LogicOutDataTypeMode=boolean
  Demux2 : Demux  Outputs=6
  Display : Display
  Display1 : Display
  Intregrator{1..5} (5 alike) : Integrator
  Intregrator6 : Integrator  ExternalReset=rising  InitialCondition=0.5
  Logical Operator : Logic  Orientation=left  Operator=OR  AllPortsSameDT=off  OutDataTypeMode=Boolean
  Mux2 : Mux  Inputs=6
  Out1 : Outport
  wires:
  Demux2/1 -> Intregrator2/1
  Demux2/2 -> Intregrator1/1
  Demux2/3 -> Intregrator3/1
  Demux2/4 -> Intregrator5/1
  Demux2/5 -> Intregrator4/1
  Intregrator2/1 -> Mux2/1
  Intregrator1/1 -> Mux2/2
  Intregrator3/1 -> Mux2/3
  Intregrator5/1 -> Mux2/4
  In1/1 -> Demux2/1
  Mux2/1 -> Out1/1
  Intregrator4/1 -> Mux2/5
  Demux2/6 -> Intregrator6/1
  Logical Operator/1 -> Intregrator6/2, Display1/1
  Compare To Constant1/1 -> Logical Operator/2
  Compare To Constant/1 -> Logical Operator/1
  Intregrator6/1 -> Display/1, Compare To Constant/1, Compare To Constant1/1, Mux2/6

== system rov_property/Euler Transformation/Transformation matrix R ==
  angular body  velocity : Inport  Port=1  LatchInput=off
  angular position : Inport  Port=2  LatchInput=off
  Mux : Mux  Inputs=3
  Row1 of T : Subsystem
      mask Display: disp('Row 1')
  Row2 of T : Subsystem
      mask Display: disp('Row 2')
  Row3 of T : Subsystem
      mask Display: disp('Row 3')
  angular earth velocity : Outport
  wires:
  angular position/1 -> Row3 of T/2(angular position), Row1 of T/2(angular position), Row2 of T/2(angular position)
  Mux/1 -> angular earth velocity/1
  Row3 of T/1(angular earth velocity (row 3)) -> Mux/3
  Row2 of T/1(angular earth velocity (row 2)) -> Mux/2
  Row1 of T/1(angular earth velocity (row 1)) -> Mux/1
  angular body  velocity/1 -> Row3 of T/1("angular body velocity "), Row2 of T/1("angular body velocity "), Row1 of T/1(angular body  velocity)

== system rov_property/Euler Transformation/Transformation matrix T ==
  translational body velocity : Inport  Port=1  LatchInput=off
  angular position : Inport  Port=2  LatchInput=off
  Mux : Mux  Inputs=3
  Row1 of R : Subsystem
      mask Display: disp('Row 1')
  Row2 of R : Subsystem
      mask Display: disp('Row 2')
  Row3 of R : Subsystem
      mask Display: disp('Row 3')
  translational earth velocity : Outport  InitialOutput=0
  wires:
  Mux/1 -> translational earth velocity/1
  Row3 of R/1(translational earth velocity (row 3)) -> Mux/3
  Row2 of R/1(translational earth velocity (row 2)) -> Mux/2
  Row1 of R/1(translational earth velocity (row 1)) -> Mux/1
  angular position/1 -> Row3 of R/2(angular position), Row1 of R/2(angular position), Row2 of R/2(angular position)
  translational body velocity/1 -> Row1 of R/1(translational body velocity), Row2 of R/1(translational body velocity), Row3 of R/1(translational body velocity)

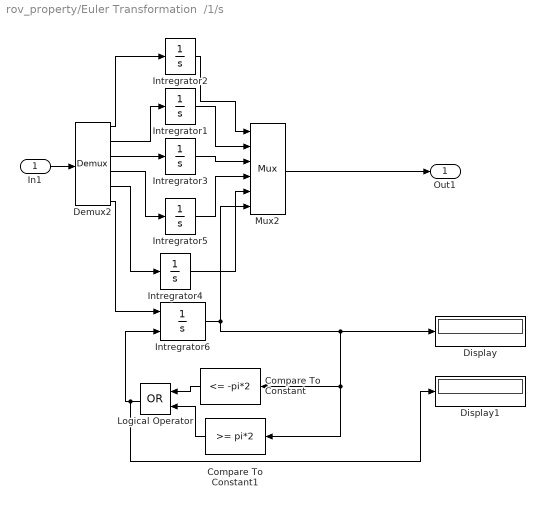
== system rov_property/Euler Transformation  /1/s ==
  In1 : Inport  Port=1  LatchInput=off
  Compare To Constant : simulink/Logic and Bit Operations/Compare To Constant  Orientation=left  relop=<=  const=-pi*2  LogicOutDataTypeMode=boolean
  Compare To Constant1 : simulink/Logic and Bit Operations/Compare To Constant  Orientation=left  relop=>=  const=pi*2  LogicOutDataTypeMode=boolean
  Demux2 : Demux  Outputs=6
  Display : Display
  Display1 : Display
  Intregrator{1..5} (5 alike) : Integrator
  Intregrator6 : Integrator  ExternalReset=rising  InitialCondition=0.5
  Logical Operator : Logic  Orientation=left  Operator=OR  AllPortsSameDT=off  OutDataTypeMode=Boolean
  Mux2 : Mux  Inputs=6
  Out1 : Outport
  wires:
  Demux2/1 -> Intregrator2/1
  Demux2/2 -> Intregrator1/1
  Demux2/3 -> Intregrator3/1
  Demux2/4 -> Intregrator5/1
  Demux2/5 -> Intregrator4/1
  Intregrator2/1 -> Mux2/1
  Intregrator1/1 -> Mux2/2
  Intregrator3/1 -> Mux2/3
  Intregrator5/1 -> Mux2/4
  In1/1 -> Demux2/1
  Mux2/1 -> Out1/1
  Intregrator4/1 -> Mux2/5
  Demux2/6 -> Intregrator6/1
  Logical Operator/1 -> Intregrator6/2, Display1/1
  Compare To Constant1/1 -> Logical Operator/2
  Compare To Constant/1 -> Logical Operator/1
  Intregrator6/1 -> Display/1, Compare To Constant/1, Compare To Constant1/1, Mux2/6

== system rov_property/Euler Transformation  /Transformation matrix R ==
  angular body  velocity : Inport  Port=1  LatchInput=off
  angular position : Inport  Port=2  LatchInput=off
  Mux : Mux  Inputs=3
  Row1 of T : Subsystem
      mask Display: disp('Row 1')
  Row2 of T : Subsystem
      mask Display: disp('Row 2')
  Row3 of T : Subsystem
      mask Display: disp('Row 3')
  angular earth velocity : Outport
  wires:
  angular position/1 -> Row3 of T/2(angular position), Row1 of T/2(angular position), Row2 of T/2(angular position)
  Mux/1 -> angular earth velocity/1
  Row3 of T/1(angular earth velocity (row 3)) -> Mux/3
  Row2 of T/1(angular earth velocity (row 2)) -> Mux/2
  Row1 of T/1(angular earth velocity (row 1)) -> Mux/1
  angular body  velocity/1 -> Row3 of T/1("angular body velocity "), Row2 of T/1("angular body velocity "), Row1 of T/1(angular body  velocity)

== system rov_property/Euler Transformation  /Transformation matrix T ==
  translational body velocity : Inport  Port=1  LatchInput=off
  angular position : Inport  Port=2  LatchInput=off
  Mux : Mux  Inputs=3
  Row1 of R : Subsystem
      mask Display: disp('Row 1')
  Row2 of R : Subsystem
      mask Display: disp('Row 2')
  Row3 of R : Subsystem
      mask Display: disp('Row 3')
  translational earth velocity : Outport  InitialOutput=0
  wires:
  Mux/1 -> translational earth velocity/1
  Row3 of R/1(translational earth velocity (row 3)) -> Mux/3
  Row2 of R/1(translational earth velocity (row 2)) -> Mux/2
  Row1 of R/1(translational earth velocity (row 1)) -> Mux/1
  angular position/1 -> Row3 of R/2(angular position), Row1 of R/2(angular position), Row2 of R/2(angular position)
  translational body velocity/1 -> Row1 of R/1(translational body velocity), Row2 of R/1(translational body velocity), Row3 of R/1(translational body velocity)

== system rov_property/Euler Transformation/Transformation matrix R/Row1 of T ==
  angular body  velocity : Inport  Port=1  LatchInput=off
  angular position : Inport  Port=2  LatchInput=off
  1 : Fcn  Expr=1
  Dot Product1 : simulink/Math Operations/Dot Product  InputSameDT=on  OutDataType=sfix(16)  OutScaling=2^-10  DoSatur=off
  Mux1 : Mux  Inputs=3
  cX.tY : Fcn  Expr=cos(u[1])*tan(u[2])
  sX.tY : Fcn  Expr=sin(u[1])*tan(u[2])
  angular earth velocity (row 1) : Outport
  wires:
  Dot Product1/1 -> angular earth velocity (row 1)/1
  angular body  velocity/1 -> Dot Product1/2
  Mux1/1 -> Dot Product1/1
  cX.tY/1 -> Mux1/3
  sX.tY/1 -> Mux1/2
  1/1 -> Mux1/1
  angular position/1 -> cX.tY/1, sX.tY/1, 1/1

== system rov_property/Euler Transformation/Transformation matrix R/Row2 of T ==
  "angular body velocity " : Inport  Port=1  LatchInput=off
  angular position : Inport  Port=2  LatchInput=off
  -sX : Fcn  Expr=-sin(u[1])
  0 : Fcn  Expr=0
  Dot Product1 : simulink/Math Operations/Dot Product  InputSameDT=on  OutDataType=sfix(16)  OutScaling=2^-10  DoSatur=off
  Mux1 : Mux  Inputs=3
  cX : Fcn  Expr=cos(u[1])
  angular earth velocity (row 2) : Outport
  wires:
  Dot Product1/1 -> angular earth velocity (row 2)/1
  "angular body velocity "/1 -> Dot Product1/2
  Mux1/1 -> Dot Product1/1
  -sX/1 -> Mux1/3
  cX/1 -> Mux1/2
  0/1 -> Mux1/1
  angular position/1 -> -sX/1, cX/1, 0/1

== system rov_property/Euler Transformation/Transformation matrix R/Row3 of T ==
  "angular body velocity " : Inport  Port=1  LatchInput=off
  angular position : Inport  Port=2  LatchInput=off
  1 : Fcn  Expr=0
  Dot Product1 : simulink/Math Operations/Dot Product  InputSameDT=on  OutDataType=sfix(16)  OutScaling=2^-10  DoSatur=off
  Mux1 : Mux  Inputs=3
  cX/cY : Fcn  Expr=cos(u[1])/cos(u[2])
  sX/cY : Fcn  Expr=sin(u[1])/cos(u[2])
  angular earth velocity (row 3) : Outport
  wires:
  Dot Product1/1 -> angular earth velocity (row 3)/1
  "angular body velocity "/1 -> Dot Product1/2
  Mux1/1 -> Dot Product1/1
  cX/cY/1 -> Mux1/3
  sX/cY/1 -> Mux1/2
  1/1 -> Mux1/1
  angular position/1 -> cX/cY/1, sX/cY/1, 1/1

== system rov_property/Euler Transformation/Transformation matrix T/Row1 of R ==
  translational body velocity : Inport  Port=1  LatchInput=off
  angular position : Inport  Port=2  LatchInput=off
  -sZ.cX+cZ.sY.sX : Fcn  Expr=-sin(u[3])*cos(u[1]) + cos(u[3])*sin(u[2])*sin(u[1])
  Dot Product : simulink/Math Operations/Dot Product  InputSameDT=on  OutDataType=sfix(16)  OutScaling=2^-10  DoSatur=off
  Mux : Mux  Inputs=3
  cY.cZ : Fcn  Expr=cos(u[3]) * cos(u[2])
  sZ.sX+cZ.cX.sY : Fcn  Expr=sin(u[3])*sin(u[1]) + cos(u[3])*cos(u[1])*sin(u[2])
  translational earth velocity (row 1) : Outport
  wires:
  Dot Product/1 -> translational earth velocity (row 1)/1
  translational body velocity/1 -> Dot Product/2
  Mux/1 -> Dot Product/1
  sZ.sX+cZ.cX.sY/1 -> Mux/3
  -sZ.cX+cZ.sY.sX/1 -> Mux/2
  cY.cZ/1 -> Mux/1
  angular position/1 -> sZ.sX+cZ.cX.sY/1, -sZ.cX+cZ.sY.sX/1, cY.cZ/1

== system rov_property/Euler Transformation/Transformation matrix T/Row2 of R ==
  translational body velocity : Inport  Port=1  LatchInput=off
  angular position : Inport  Port=2  LatchInput=off
  -cZ.sX+sY.sZ.cX : Fcn  Expr=-cos(u[3])*sin(u[1]) + sin(u[2])*sin(u[3])*cos(u[1])
  Dot Product1 : simulink/Math Operations/Dot Product  InputSameDT=on  OutDataType=sfix(16)  OutScaling=2^-10  DoSatur=off
  Mux1 : Mux  Inputs=3
  cY.sZ : Fcn  Expr=sin(u[3]) * cos(u[2])
  cZ.cX+sX.sY.sZ : Fcn  Expr=cos(u[3])*cos(u[1]) + sin(u[1])*sin(u[2])*sin(u[3])
  translational earth velocity (row 2) : Outport
  wires:
  Dot Product1/1 -> translational earth velocity (row 2)/1
  translational body velocity/1 -> Dot Product1/2
  Mux1/1 -> Dot Product1/1
  -cZ.sX+sY.sZ.cX/1 -> Mux1/3
  cZ.cX+sX.sY.sZ/1 -> Mux1/2
  cY.sZ/1 -> Mux1/1
  angular position/1 -> -cZ.sX+sY.sZ.cX/1, cZ.cX+sX.sY.sZ/1, cY.sZ/1

== system rov_property/Euler Transformation/Transformation matrix T/Row3 of R ==
  translational body velocity : Inport  Port=1  LatchInput=off
  angular position : Inport  Port=2  LatchInput=off
  -sY : Fcn  Expr=-sin(u[2])
  Dot Product1 : simulink/Math Operations/Dot Product  InputSameDT=on  OutDataType=sfix(16)  OutScaling=2^-10  DoSatur=off
  Mux1 : Mux  Inputs=3
  cY.cX : Fcn  Expr=cos(u[2])*cos(u[1])
  cY.sX : Fcn  Expr=cos(u[2])*sin(u[1])
  translational earth velocity (row 3) : Outport  InitialOutput=0
  wires:
  Dot Product1/1 -> translational earth velocity (row 3)/1
  translational body velocity/1 -> Dot Product1/2
  Mux1/1 -> Dot Product1/1
  cY.cX/1 -> Mux1/3
  cY.sX/1 -> Mux1/2
  -sY/1 -> Mux1/1
  angular position/1 -> cY.cX/1, cY.sX/1, -sY/1

== system rov_property/Euler Transformation  /Transformation matrix R/Row1 of T ==
  angular body  velocity : Inport  Port=1  LatchInput=off
  angular position : Inport  Port=2  LatchInput=off
  1 : Fcn  Expr=1
  Dot Product1 : simulink/Math Operations/Dot Product  InputSameDT=on  OutDataType=sfix(16)  OutScaling=2^-10  DoSatur=off
  Mux1 : Mux  Inputs=3
  cX.tY : Fcn  Expr=cos(u[1])*tan(u[2])
  sX.tY : Fcn  Expr=sin(u[1])*tan(u[2])
  angular earth velocity (row 1) : Outport
  wires:
  Dot Product1/1 -> angular earth velocity (row 1)/1
  angular body  velocity/1 -> Dot Product1/2
  Mux1/1 -> Dot Product1/1
  cX.tY/1 -> Mux1/3
  sX.tY/1 -> Mux1/2
  1/1 -> Mux1/1
  angular position/1 -> cX.tY/1, sX.tY/1, 1/1

== system rov_property/Euler Transformation  /Transformation matrix R/Row2 of T ==
  "angular body velocity " : Inport  Port=1  LatchInput=off
  angular position : Inport  Port=2  LatchInput=off
  -sX : Fcn  Expr=-sin(u[1])
  0 : Fcn  Expr=0
  Dot Product1 : simulink/Math Operations/Dot Product  InputSameDT=on  OutDataType=sfix(16)  OutScaling=2^-10  DoSatur=off
  Mux1 : Mux  Inputs=3
  cX : Fcn  Expr=cos(u[1])
  angular earth velocity (row 2) : Outport
  wires:
  Dot Product1/1 -> angular earth velocity (row 2)/1
  "angular body velocity "/1 -> Dot Product1/2
  Mux1/1 -> Dot Product1/1
  -sX/1 -> Mux1/3
  cX/1 -> Mux1/2
  0/1 -> Mux1/1
  angular position/1 -> -sX/1, cX/1, 0/1

== system rov_property/Euler Transformation  /Transformation matrix R/Row3 of T ==
  "angular body velocity " : Inport  Port=1  LatchInput=off
  angular position : Inport  Port=2  LatchInput=off
  1 : Fcn  Expr=0
  Dot Product1 : simulink/Math Operations/Dot Product  InputSameDT=on  OutDataType=sfix(16)  OutScaling=2^-10  DoSatur=off
  Mux1 : Mux  Inputs=3
  cX/cY : Fcn  Expr=cos(u[1])/cos(u[2])
  sX/cY : Fcn  Expr=sin(u[1])/cos(u[2])
  angular earth velocity (row 3) : Outport
  wires:
  Dot Product1/1 -> angular earth velocity (row 3)/1
  "angular body velocity "/1 -> Dot Product1/2
  Mux1/1 -> Dot Product1/1
  cX/cY/1 -> Mux1/3
  sX/cY/1 -> Mux1/2
  1/1 -> Mux1/1
  angular position/1 -> cX/cY/1, sX/cY/1, 1/1

== system rov_property/Euler Transformation  /Transformation matrix T/Row1 of R ==
  translational body velocity : Inport  Port=1  LatchInput=off
  angular position : Inport  Port=2  LatchInput=off
  -sZ.cX+cZ.sY.sX : Fcn  Expr=-sin(u[3])*cos(u[1]) + cos(u[3])*sin(u[2])*sin(u[1])
  Dot Product : simulink/Math Operations/Dot Product  InputSameDT=on  OutDataType=sfix(16)  OutScaling=2^-10  DoSatur=off
  Mux : Mux  Inputs=3
  cY.cZ : Fcn  Expr=cos(u[3]) * cos(u[2])
  sZ.sX+cZ.cX.sY : Fcn  Expr=sin(u[3])*sin(u[1]) + cos(u[3])*cos(u[1])*sin(u[2])
  translational earth velocity (row 1) : Outport
  wires:
  Dot Product/1 -> translational earth velocity (row 1)/1
  translational body velocity/1 -> Dot Product/2
  Mux/1 -> Dot Product/1
  sZ.sX+cZ.cX.sY/1 -> Mux/3
  -sZ.cX+cZ.sY.sX/1 -> Mux/2
  cY.cZ/1 -> Mux/1
  angular position/1 -> sZ.sX+cZ.cX.sY/1, -sZ.cX+cZ.sY.sX/1, cY.cZ/1
